simulink model "two_buck_DQN"  (R2022b)
settings: Solver=VariableStepAuto  StartTime=0.0  StopTime=0.5  RelTol=1e-3
undefined symbols (not defined in the file or in its folder): R
libraries: spsSeriesRLCBranchLib x7, spsCurrentMeasurementLib x4, simulink x3, spsPWMGeneratorDCDCLib x2, spsControlledVoltageSourceLib x2, spsDiodeLib x2, spsMosfetLib x2, rllib x1, spsControlledCurrentSourceLib x1, spsVoltageMeasurementLib x1, spspowerguiLib x1
settings Model: Creator=Sweet_J  LastModifiedBy=Sweet_J

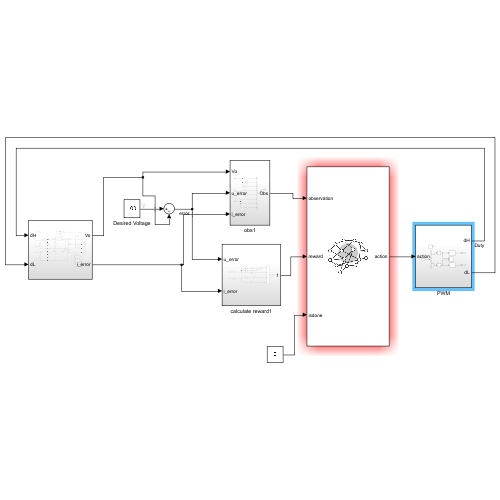
[thumbnail: Simulink's stored preview of the top-level diagram]
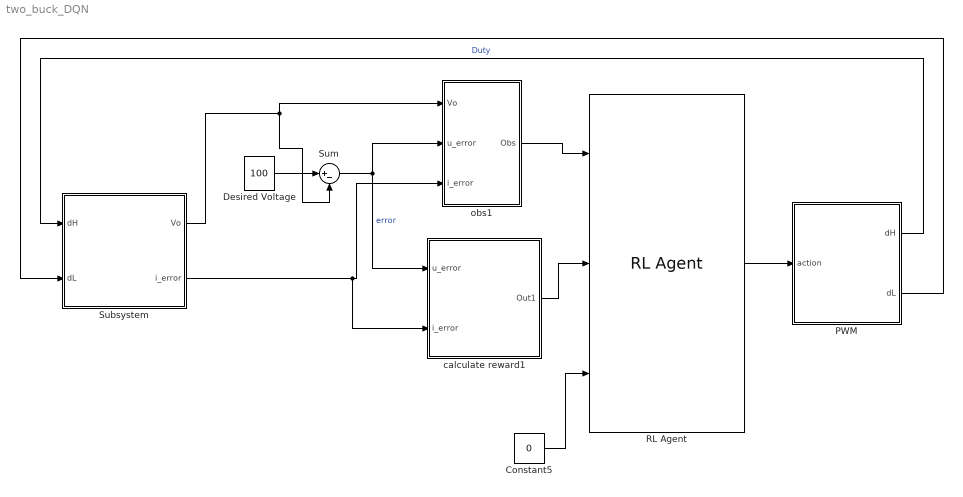
== system two_buck_DQN ==
  Constant5 : Constant  Value=0
  Desired Voltage : Constant  Value=100
  PWM : Subsystem
  RL Agent : rllib/RL Agent  Agent=agentObj  ExternalActionAsInput=off  ProvideLastAction=off  ProvideCumRwd=off  TreatAsDirectFeedthrough=on  UseStrictObservationDataTypes=off
  Subsystem : Subsystem
  Sum : Sum  Inputs=|+-
  calculate reward1 : Subsystem
  obs1 : Subsystem
  wires:
  Sum/1 -> calculate reward1/1(u_error), obs1/2(u_error)  "error"
  obs1/1(Obs) -> RL Agent/1
  Constant5/1 -> RL Agent/3
  Desired Voltage/1 -> Sum/1
  calculate reward1/1(Out1) -> RL Agent/2
  RL Agent/1 -> PWM/1(action)
  Subsystem/1(Vo) -> Sum/2, obs1/1(Vo)
  PWM/1(dH) -> Subsystem/1(dH)  "Duty"
  PWM/2(dL) -> Subsystem/2(dL)
  Subsystem/2(i_error) -> calculate reward1/2(i_error), obs1/3(i_error)

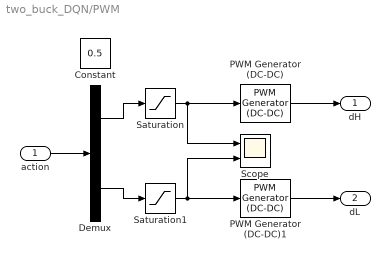
== system two_buck_DQN/PWM ==
  action : Inport
  Constant : Constant  Value=0.5
  Demux : Demux  Outputs=2
  PWM Generator (DC-DC) : spsPWMGeneratorDCDCLib/PWM Generator (DC-DC)  Fsw=10000  Ts=0
  PWM Generator (DC-DC)1 : spsPWMGeneratorDCDCLib/PWM Generator (DC-DC)  Fsw=10000  Ts=0
  Saturation : Saturate  UpperLimit=0.99  LowerLimit=0.01  ZeroCross=off
  Saturation1 : Saturate  UpperLimit=0.99  LowerLimit=0.01  ZeroCross=off
  Scope : Scope  NumInputPorts=2
  dH : Outport  VectorParamsAs1DForOutWhenUnconnected=off
  dL : Outport  Port=2
  wires:
  PWM Generator (DC-DC)/1 -> dH/1
  Saturation/1 -> Scope/1, PWM Generator (DC-DC)/1
  PWM Generator (DC-DC)1/1 -> dL/1
  Saturation1/1 -> Scope/2, PWM Generator (DC-DC)1/1
  action/1 -> Demux/1
  Demux/1 -> Saturation/1
  Demux/2 -> Saturation1/1

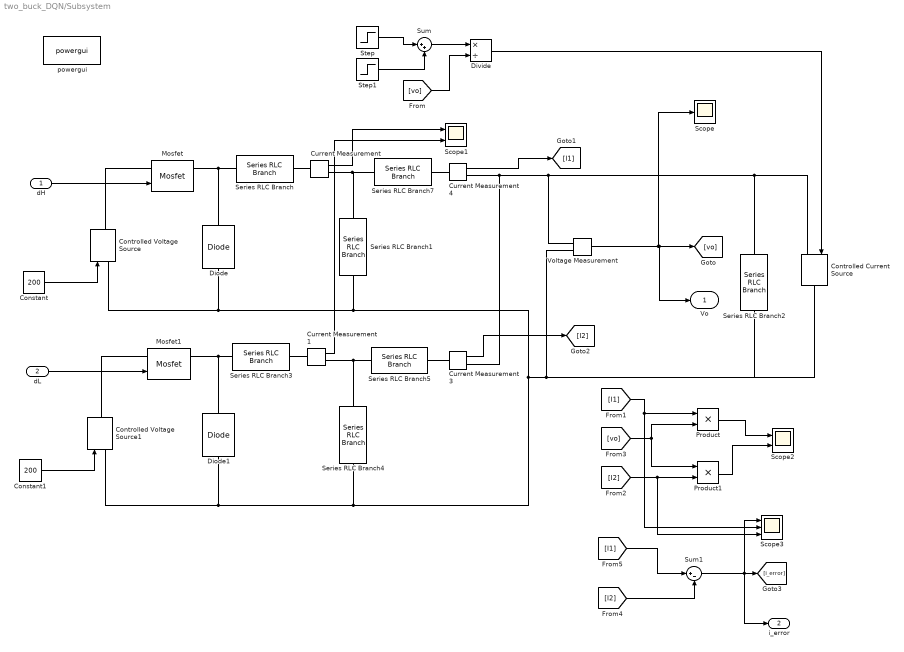
== system two_buck_DQN/Subsystem ==
  dH : Inport
  dL : Inport  Port=2
  Constant : Constant  Value=200
  Constant1 : Constant  Value=200
  Controlled Current Source : spsControlledCurrentSourceLib/Controlled Current Source  Initialize=on  Source_Type=AC  Amplitude=0  Phase=0  Frequency=0  Measurements=None
  Controlled Voltage Source : spsControlledVoltageSourceLib/Controlled Voltage Source  Initialize=on  Source_Type=AC  Amplitude=0  Phase=0  Frequency=0  Measurements=None
  Controlled Voltage Source1 : spsControlledVoltageSourceLib/Controlled Voltage Source  Initialize=on  Source_Type=AC  Amplitude=0  Phase=0  Frequency=0  Measurements=None
  Current Measurement{,1,3..4} (4 alike) : spsCurrentMeasurementLib/Current Measurement  PhasorSimulation=off  OutputType=Complex  PSBequivalent=0
  Diode : spsDiodeLib/Diode  Ron=0.001  Lon=0  Vf=0.8  IC=0  UseSnubber=0  Rs=500  Cs=250e-9  Measurements=off
  Diode1 : spsDiodeLib/Diode  Ron=0.001  Lon=0  Vf=0.8  IC=0  UseSnubber=0  Rs=500  Cs=250e-9  Measurements=off
  Divide : Product  Inputs=*/
  Mosfet : spsMosfetLib/Mosfet  Ron=0.1  Lon=0  Rd=0.01  Vfd=0  IC=0  Rs=1e5  Cs=inf  Measurements=on
  Mosfet1 : spsMosfetLib/Mosfet  Ron=0.1  Lon=0  Rd=0.01  Vfd=0  IC=0  Rs=1e5  Cs=inf  Measurements=on
  Product : Product
  Product1 : Product
  Scope : Scope
  Scope1 : Scope  NumInputPorts=2
  Scope2 : Scope  NumInputPorts=2
  Scope3 : Scope  NumInputPorts=3
  Series RLC Branch : spsSeriesRLCBranchLib/Series RLC Branch  LConnTagsString=__new0  RConnTagsString=__new0  BranchType=L  Resistance=1  Inductance=0.002  SetiL0=off  InitialCurrent=0  Capacitance=1e-6  Setx0=off  InitialVoltage=0  Measurements=None
  Series RLC Branch1 : spsSeriesRLCBranchLib/Series RLC Branch  LConnTagsString=__new0  RConnTagsString=__new0  BranchType=C  Resistance=1  Inductance=0.002  SetiL0=off  InitialCurrent=0  Capacitance=0.0015  Setx0=on  InitialVoltage=100  Measurements=None
  Series RLC Branch2 : spsSeriesRLCBranchLib/Series RLC Branch  LConnTagsString=__new0  RConnTagsString=__new0  BranchType=R  Resistance=10000  Inductance=R  SetiL0=off  InitialCurrent=0  Capacitance=1e-6  Setx0=off  InitialVoltage=0  Measurements=None
  Series RLC Branch3 : spsSeriesRLCBranchLib/Series RLC Branch  LConnTagsString=__new0  RConnTagsString=__new0  BranchType=L  Resistance=1  Inductance=0.002  SetiL0=off  InitialCurrent=0  Capacitance=1e-6  Setx0=off  InitialVoltage=0  Measurements=None
  Series RLC Branch4 : spsSeriesRLCBranchLib/Series RLC Branch  LConnTagsString=__new0  RConnTagsString=__new0  BranchType=C  Resistance=1  Inductance=0.002  SetiL0=off  InitialCurrent=0  Capacitance=0.0015  Setx0=on  InitialVoltage=100  Measurements=None
  Series RLC Branch5 : spsSeriesRLCBranchLib/Series RLC Branch  LConnTagsString=__new0  RConnTagsString=__new0  BranchType=R  Resistance=0.4  Inductance=1e-4  SetiL0=off  InitialCurrent=0  Capacitance=1e-6  Setx0=off  InitialVoltage=0  Measurements=None
  Series RLC Branch7 : spsSeriesRLCBranchLib/Series RLC Branch  LConnTagsString=__new0  RConnTagsString=__new0  BranchType=R  Resistance=0.6  Inductance=1e-4  SetiL0=off  InitialCurrent=0  Capacitance=1e-6  Setx0=off  InitialVoltage=0  Measurements=None
  Step : Step  Time=0.1  Before=300  After=800  SampleTime=0
  Step1 : Step  Time=0.3  After=-300  SampleTime=0
  Sum : Sum  Inputs=|++
  Sum1 : Sum  Inputs=|+-
  Voltage Measurement : spsVoltageMeasurementLib/Voltage Measurement  PhasorSimulation=off  OutputType=Complex  PSBequivalent=0
  powergui : spspowerguiLib/powergui  Priority=1  SimulationMode=Continuous  SampleTime=50e-6  frequency=60  Iterations=50  frequencyindice=0  Pbase=100e6  ErrMax=1e-4  UnitsV=kV  UnitsW=MW  buscounter=0  FunctionMessages=off  echomessages=off  EnableUseOfTLC=off  CurrentSourceSwitches=off  DisableSnubberDevices=off  DisableRonSwitches=off  DisableVfSwitches=off  DisplayEquations=off  AutomaticDiscreteSolvers=off  SolverType=Tustin/Backward Euler (TBE)  Interpol=off  ExternalGateDelay=off  methode=off  Ts=100  x0status=blocks  SPID=on  SwTol=0  HookPort=off  NonlinearTolerance=0  nMaxIteration=15  ContinueOnMaxIteration=off  RestoreLinks=warning  ResistiveCurrentMeasurement=off  Frange=[0:2:500]  Ylog=off  Xlog=on  ShowGrid=off  save=off  variable=ZData  structure=0  ZoomFFT=off  StartTime=0.0  cycles=1  DisplayStyle=1  fundamental=60  FreqAxis=off  MaxFrequency=1000  frequencyindicesteady=1  RmsSteady=1  display=off
  Vo : Outport  VectorParamsAs1DForOutWhenUnconnected=off
  i_error : Outport  Port=2
  wires:
  Sum/1 -> Divide/1
  [vo] -> Divide/2
  Current Measurement/1 -> Scope1/1
  Step1/1 -> Sum/2
  Step/1 -> Sum/1
  dH/1 -> Mosfet/1
  Divide/1 -> Controlled Current Source/1
  Constant/1 -> Controlled Voltage Source/1
  dL/1 -> Mosfet1/1
  Constant1/1 -> Controlled Voltage Source1/1
  Current Measurement1/1 -> Scope1/2
  Voltage Measurement/1 -> [vo], Vo/1, Scope/1
  Current Measurement4/1 -> [I1]
  Current Measurement3/1 -> [I2]
  [I1] -> Scope3/2, Product/1
  [vo] -> Product1/1, Product/2
  [I2] -> Scope3/3, Product1/2
  Product/1 -> Scope2/1
  Product1/1 -> Scope2/2
  [I1] -> Sum1/1
  [I2] -> Sum1/2
  Sum1/1 -> Scope3/1, i_error/1, [i_error]
  connections:
  Series RLC Branch4/RConn1 -- Controlled Voltage Source1/LConn1 -- Diode1/LConn1 -- Voltage Measurement/LConn2 -- Controlled Current Source/RConn1 -- Series RLC Branch2/RConn1 -- Diode/LConn1 -- Controlled Voltage Source/LConn1 -- Series RLC Branch1/RConn1
  Diode/RConn1 -- Series RLC Branch/LConn1 -- Mosfet/RConn1
  Mosfet/LConn1 -- Controlled Voltage Source/RConn1
  Series RLC Branch/RConn1 -- Current Measurement/LConn1
  Mosfet1/RConn1 -- Diode1/RConn1 -- Series RLC Branch3/LConn1
  Mosfet1/LConn1 -- Controlled Voltage Source1/RConn1
  Series RLC Branch3/RConn1 -- Current Measurement1/LConn1
  Series RLC Branch7/LConn1 -- Current Measurement/RConn1 -- Series RLC Branch1/LConn1
  Current Measurement1/RConn1 -- Series RLC Branch5/LConn1 -- Series RLC Branch4/LConn1
  Current Measurement3/RConn1 -- Controlled Current Source/LConn1 -- Series RLC Branch2/LConn1 -- Voltage Measurement/LConn1 -- Current Measurement4/RConn1
  Current Measurement4/LConn1 -- Series RLC Branch7/RConn1
  Current Measurement3/LConn1 -- Series RLC Branch5/RConn1

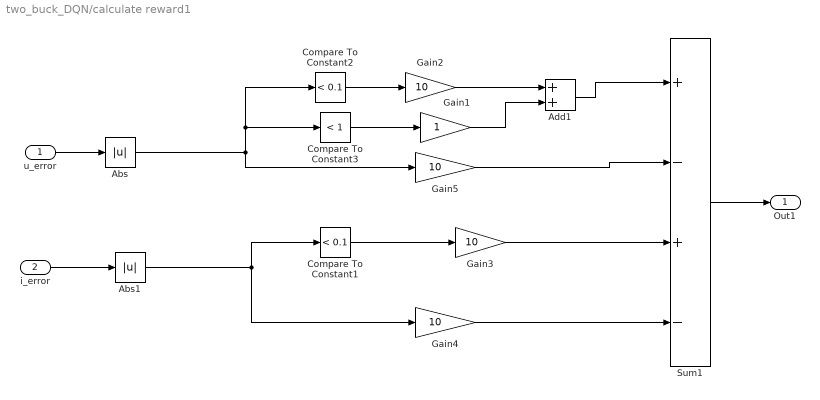
== system two_buck_DQN/calculate reward1 ==
  u_error : Inport
  i_error : Inport  Port=2
  Abs : Abs  ZeroCross=off  SaturateOnIntegerOverflow=off
  Abs1 : Abs  ZeroCross=off  SaturateOnIntegerOverflow=off
  Add1 : Sum
  Compare To Constant1 : simulink/Logic and Bit Operations/Compare To Constant  relop=<  const=0.1  OutDataTypeStr=boolean  ZeroCross=off
  Compare To Constant2 : simulink/Logic and Bit Operations/Compare To Constant  relop=<  const=0.1  OutDataTypeStr=boolean  ZeroCross=off
  Compare To Constant3 : simulink/Logic and Bit Operations/Compare To Constant  relop=<  const=1  OutDataTypeStr=boolean  ZeroCross=off
  Gain1 : Gain
  Gain{2..5} (4 alike) : Gain  Gain=10
  Sum1 : Sum  Inputs=+-+-  OutDataTypeStr=double
  Out1 : Outport
  wires:
  u_error/1 -> Abs/1
  Compare To Constant2/1 -> Gain2/1
  Gain5/1 -> Sum1/2
  Gain2/1 -> Add1/1
  Add1/1 -> Sum1/1
  Abs/1 -> Gain5/1, Compare To Constant2/1, Compare To Constant3/1
  Compare To Constant3/1 -> Gain1/1
  Gain1/1 -> Add1/2
  Sum1/1 -> Out1/1
  i_error/1 -> Abs1/1
  Abs1/1 -> Gain4/1, Compare To Constant1/1
  Compare To Constant1/1 -> Gain3/1
  Gain4/1 -> Sum1/4
  Gain3/1 -> Sum1/3

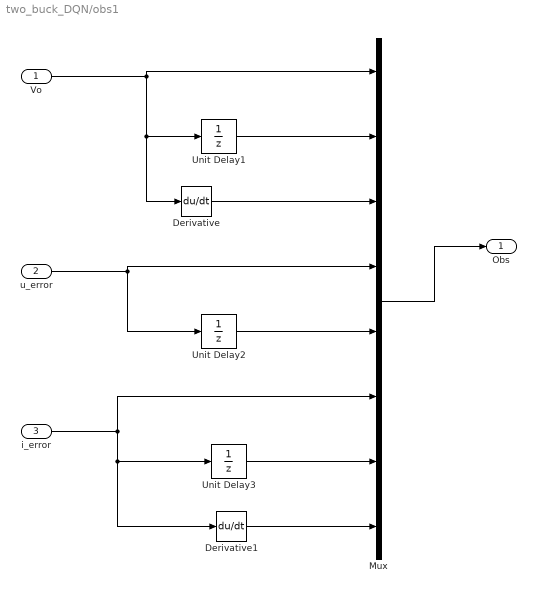
== system two_buck_DQN/obs1 ==
  Vo : Inport
  u_error : Inport  Port=2
  i_error : Inport  Port=3
  Derivative : Derivative
  Derivative1 : Derivative
  Mux : Mux  Inputs=8
  Unit Delay1 : UnitDelay  SampleTime=-1  HasFrameUpgradeWarning=on
  Unit Delay2 : UnitDelay  SampleTime=-1  HasFrameUpgradeWarning=on
  Unit Delay3 : UnitDelay  SampleTime=-1  HasFrameUpgradeWarning=on
  Obs : Outport
  wires:
  u_error/1 -> Unit Delay2/1, Mux/4
  Mux/1 -> Obs/1
  Derivative/1 -> Mux/3
  Vo/1 -> Mux/1, Derivative/1, Unit Delay1/1
  Unit Delay1/1 -> Mux/2
  Unit Delay2/1 -> Mux/5
  i_error/1 -> Mux/6, Derivative1/1, Unit Delay3/1
  Unit Delay3/1 -> Mux/7
  Derivative1/1 -> Mux/8
